simulink model "RoboSoccer"
settings: Solver=ode15s  StartTime=0.0  StopTime=inf  RelTol=1e-3
PreLoadFcn:
  | load busobjects.mat;
libraries: simulink x5
settings Model: Creator=smahapat  LastModifiedBy=user
settings SolverCC: ZeroCrossControl=DisableAll
settings DataIOCC: LimitDataPoints=on  SaveFormat=Array  SignalLoggingSaveFormat=ModelDataLogs  ReturnWorkspaceOutputs=off
settings OptimizationCC: InlineParams=on  ExpressionDepthLimit=2147483647  LifeSpan=inf  SimCompilerOptimization=Off
settings DebuggingCC: UnderspecifiedInitializationDetection=Classic  MergeDetectMultiDrivingBlocksExec=none  SolverPrmCheckMsg=warning  FcnCallInpInsideContextMsg=Use local settings  FrameProcessingCompatibilityMsg=warning  StateNameClashWarn=warning  SFUnexpectedBacktrackingDiag=warning  SFNoUnconditionalDefaultTransitionDiag=warning
settings HardwareCC: ProdBitPerPointer=32  ProdLargestAtomicFloat=None  ProdIntDivRoundTo=Undefined  ProdEndianess=Unspecified  ProdWordSize=32  ProdHWDeviceType=32-bit Generic
settings ModelReferenceCC: PropagateSignalLabelsOutOfModel=off
settings SFSimCC: SimUseLocalCustomCode=off  SimParseCustomCode=off
settings RTWCC: RTWUseLocalCustomCode=off  RTWCompilerOptimization=Off
settings CodeAppCC: CustomSymbolStrType=$N$R$M
settings GRTTargetCC: CodeReplacementLibrary=ANSI_C  GeneratePreprocessorConditionals=Disable all  CombineOutputUpdateFcns=off  CPPClassGenCompliant=off  GRTInterface=on

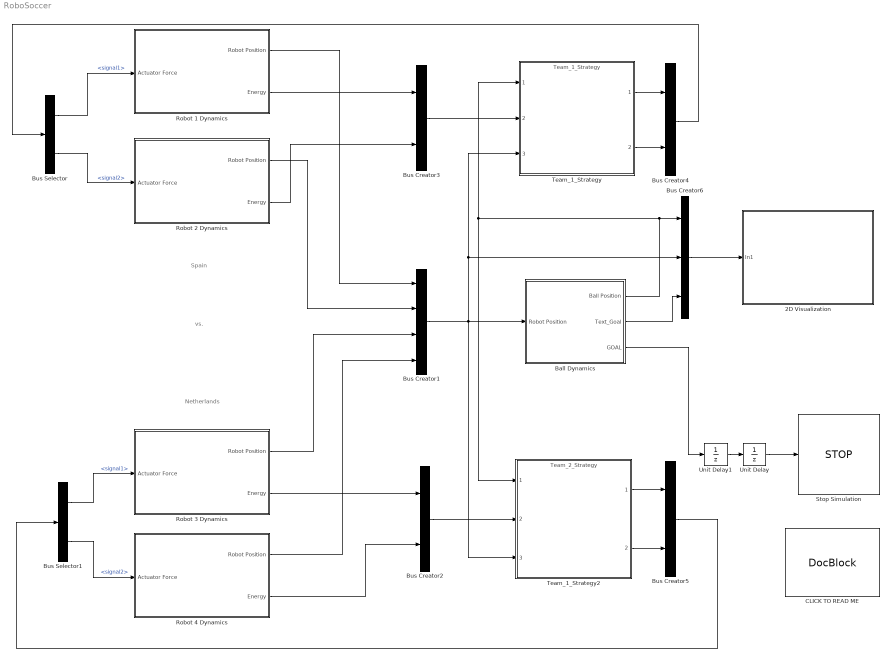
== system RoboSoccer ==
  note: Netherlands
  note: Spain
  note: vs.
  2D Visualization : Subsystem
      mask Display: image(imread('texture\3D_visualization.jpg'));
  Ball Dynamics : Subsystem  TreatAsAtomicUnit=on
      mask Display: image(imread('texture\soccer_ball_dynamics.jpg'));
  Bus Creator1 : BusCreator
  Bus Creator{2..5} (4 alike) : BusCreator  Inputs=2
  Bus Creator6 : BusCreator  Inputs=3
  Bus Selector : BusSelector  OutputSignals=signal1,signal2
  Bus Selector1 : BusSelector  OutputSignals=signal1,signal2
  CLICK TO READ ME : simulink/Model-Wide Utilities/DocBlock  DocumentType=Text
      content=|
      | Notes and help:
      | 1. The demo simulates a 2 vs. 2 robot scenario. The robots are assumed to be heavier than the football. Thus,
      | any collision between the ball and the robots is perfectly elastic. The robot motion is not impacted by the
      | collision.
      |
      | 2. Collision among robots is not implemented as they are considered as point masses.
      |
      | 3. Collision modeling in all cases is assumed to be as a spring contact model. When the object colliding with
      | a boundary comes close to that boundary, a force proprtional to the negative of the "penetration distance" is
      | computed.
      |
      | 4. The strategy subsystems are implemented as model references. This was done intentionally so that
      | competing teams could protect their strategies and run the simulation against each other. Use the model
      | protected mode to generate mdlp files instead of mdl files:
      |
      | >> Simulink.ModelReference.protect('Team_1_Strategy')
      |
      | and
      |
      | >> Simulink.ModelReference.protect('Team_2_Strategy')
      |
      | 5. Robot dynamics are simple dynamics of a point mass. However, the mass is inversely proportional to the
      | battery power or "stamina" of the robot. Some damping is also put into the system to avoid too much
      | overshoot. Also, each time the robot actuates itself or brakes, it incurs a small power loss thereby
      | lowering its endurance in the game.
      |
      | 6. Positional coordinates in the system are 2D i.e. (x,y). The signal dimensions have been set explicitly.
      | Click on any of the output ports->signal attributes of the masked subsystems to see the dimensions.
      |
      | 7. Ball dynamics has a simple implementation- same "spring-based" contact dynamics. From the ball's
      | point of view, there are five contact forces to be accounted for: contacts with the 4 robots and those of
      | the boundaries.
      |
      | 8. Observe that the solver has been changed to ode15s which is a stiff solver. The reason for this is
      | the stiffness present in the system because of the contact/collision modeling with high spring constants.
      | This can give rise to modes with relatively different dynamics. With a ode45 solver, the faster modes
      | will force the adaptive solver to take smaller steps slowing the simulation down. ode15s ignores some of
      | these fast dynamics.
      |
      | 9. All the icon drawing commands on the robot dynamics were implemented using the patch commands. These
      | were taken from the demo by Mike Woodward:
      |
      | http://www.mathworks.com/matlabcentral/fileexchange/8856-flags
      |
      | Use other flags to customize this.
      |
      | 10. 2D animation was done using Simulink 3D Animation. The field was textured with a grass image and a
      | viewpoint was so selected so that it looked as 2D. The "GOAL" text was kept behind the field. The moment,
      | a goal is scored, this text kis translated to the front giving a TV effect. Texturing was also used to
      | paint the bodies of the robots with the flags. You will have to change the images in order to change
      | these.
      |
      | 11. Play around with the strategy subsystems to see if you can come up with efficient strategies to score
      | early. Note that each of the teams has full knowledge of the others' positions and those of the ball. They
      | also have knowledge of the remaining power in their team's batteries. There is no velocity information
      | available.
      |
      | Questions:
      | 1. How can you use Stateflow to implement a fine state machine that uses a mix of attack and defensive
      | strategies based on ball location?
      |
      | 2. What block in Simulink should you use to input a new signal into these strategy subsystems so that
      | time elapsed since the start of the game can be measured and hence used as part of the strategy.
      |
      | 3. Identify the contents inside the MAT file used in the demo. What is the "type" of the contents of the
      | data inside the file? Identify the function that loads this MAT file.
      |
      | 4. Why did we need these data objects that you identified in 14 for our model?
      |
      | 5. Identify a model architecture that supports a 2n vs 2n game scenario ('n' is a natural number)
      |
      |
      |
      | 16.
  Robot 1 Dynamics : Subsystem  mask(Robot Parameters){P=0.5, saturate_value=0}
      mask prompts: P "Stamina (Enter value between 0 and 1)"; saturate_value "Actuator_saturation"
      mask help:
      | Set the robot stamina to a value between 0.1 and 1. Note that a higher value of stamina corresponds to more battery power which inversely impacts the mass of the robot. This will reduce its agility.
      |
      | Likewise, higher values of accuracy will come at a cost of higher rates of discharge for the battery pack.
      |
      | Choose values carefully to reflect these tradeoffs.
      mask init:
      | saturate_value=300;
      settings: CloseFcn=|
      | if P<0
      |     error('P cannot be less than 0');
      | end
      | if P>1
      |     error('P cannot be greater than 1');
      | end
      | 
      | if sigma<0
      |     error('sigma cannot be less than 0');
      | end
      | 
      | if sigma>1
      |     error('sigma cannot be greater than 1');
      | end
      mask Help:
      | Set the robot stamina to a value between 0.1 and 1. Note that a higher value of stamina corresponds to more battery power which inversely impacts the mass of the robot. This will reduce its agility.
      | 
      | Likewise, higher values of accuracy will come at a cost of higher rates of discharge for the battery pack.
      | 
      | Choose values carefully to reflect these tradeoffs.
      mask CallbackString: |saturate_value=10;
      mask Display:
      | patch([0 1 1 0], [0.75 0.75 1   1  ], [1 0 0]);
      | patch([0 1 1 0], [0.25 0.25 0.75 0.75], [1 1 0]);
      | patch([0 1 1 0], [0   0   0.25 0.25], [1 0 0]);
  Robot 2 Dynamics : Subsystem  mask(Robot Parameters){P=0.5, saturate_value=0}
      mask prompts: P "Stamina (Enter value between 0 and 1)"; saturate_value "Actuator_saturation"
      mask help:
      | Set the robot stamina to a value between 0.1 and 1. Note that a higher value of stamina corresponds to more battery power which inversely impacts the mass of the robot. This will reduce its agility.
      |
      | Likewise, higher values of accuracy will come at a cost of higher rates of discharge for the battery pack.
      |
      | Choose values carefully to reflect these tradeoffs.
      mask init:
      | saturate_value=300;
      settings: CloseFcn=|
      | if P<0
      |     error('P cannot be less than 0');
      | end
      | if P>1
      |     error('P cannot be greater than 1');
      | end
      | 
      | if sigma<0
      |     error('sigma cannot be less than 0');
      | end
      | 
      | if sigma>1
      |     error('sigma cannot be greater than 1');
      | end
      mask Help:
      | Set the robot stamina to a value between 0.1 and 1. Note that a higher value of stamina corresponds to more battery power which inversely impacts the mass of the robot. This will reduce its agility.
      | 
      | Likewise, higher values of accuracy will come at a cost of higher rates of discharge for the battery pack.
      | 
      | Choose values carefully to reflect these tradeoffs.
      mask CallbackString: |saturate_value=10;
      mask Display:
      | patch([0 1 1 0], [0.75 0.75 1   1  ], [1 0 0]);
      | patch([0 1 1 0], [0.25 0.25 0.75 0.75], [1 1 0]);
      | patch([0 1 1 0], [0   0   0.25 0.25], [1 0 0]);
  Robot 3 Dynamics : Subsystem  mask(Robot Parameters){P=0.5, saturate_value=0}
      mask prompts: P "Stamina (Enter value between 0 and 1)"; saturate_value "Actuator_saturation"
      mask help:
      | Set the robot stamina to a value between 0.1 and 1. Note that a higher value of stamina corresponds to more battery power which inversely impacts the mass of the robot. This will reduce its agility.
      |
      | Likewise, higher values of accuracy will come at a cost of higher rates of discharge for the battery pack.
      |
      | Choose values carefully to reflect these tradeoffs.
      mask init:
      | saturate_value=300;
      settings: CloseFcn=|
      | if P<0
      |     error('P cannot be less than 0');
      | end
      | if P>1
      |     error('P cannot be greater than 1');
      | end
      | 
      | if sigma<0
      |     error('sigma cannot be less than 0');
      | end
      | 
      | if sigma>1
      |     error('sigma cannot be greater than 1');
      | end
      mask Help:
      | Set the robot stamina to a value between 0.1 and 1. Note that a higher value of stamina corresponds to more battery power which inversely impacts the mass of the robot. This will reduce its agility.
      | 
      | Likewise, higher values of accuracy will come at a cost of higher rates of discharge for the battery pack.
      | 
      | Choose values carefully to reflect these tradeoffs.
      mask CallbackString: |saturate_value=10;
      mask Display:
      | patch([0 1 1 0], [2/3 2/3 1   1  ], [1 0 0]);
      | patch([0 1 1 0], [0   0   1/3 1/3], [0 0 1]);
  Robot 4 Dynamics : Subsystem  mask(Robot Parameters){P=0.5, saturate_value=0}
      mask prompts: P "Stamina (Enter value between 0 and 1)"; saturate_value "Actuator_saturation"
      mask help:
      | Set the robot stamina to a value between 0.1 and 1. Note that a higher value of stamina corresponds to more battery power which inversely impacts the mass of the robot. This will reduce its agility.
      |
      | Likewise, higher values of accuracy will come at a cost of higher rates of discharge for the battery pack.
      |
      | Choose values carefully to reflect these tradeoffs.
      mask init:
      | saturate_value=300;
      settings: CloseFcn=|
      | if P<0
      |     error('P cannot be less than 0');
      | end
      | if P>1
      |     error('P cannot be greater than 1');
      | end
      | 
      | if sigma<0
      |     error('sigma cannot be less than 0');
      | end
      | 
      | if sigma>1
      |     error('sigma cannot be greater than 1');
      | end
      mask Help:
      | Set the robot stamina to a value between 0.1 and 1. Note that a higher value of stamina corresponds to more battery power which inversely impacts the mass of the robot. This will reduce its agility.
      | 
      | Likewise, higher values of accuracy will come at a cost of higher rates of discharge for the battery pack.
      | 
      | Choose values carefully to reflect these tradeoffs.
      mask CallbackString: |saturate_value=10;
      mask Display:
      | patch([0 1 1 0], [2/3 2/3 1   1  ], [1 0 0]);
      | patch([0 1 1 0], [0   0   1/3 1/3], [0 0 1]);
  Stop Simulation : Stop
  Team_1_Strategy : ModelReference  ModelNameDialog=Team_1_Strategy  SimulationMode=Normal  ModelReferenceVersion=1.30  CopyOfModelName=Team_1_Strategy  DefaultDataLogging=off
      mask Display:
      | disp(' TEAM 1\n\n')
      | disp('STRATEGY')
  Team_1_Strategy2 : ModelReference  ModelNameDialog=Team_2_Strategy  SimulationMode=Normal  ModelReferenceVersion=1.28  CopyOfModelName=Team_2_Strategy  DefaultDataLogging=off
      mask Display:
      | disp(' TEAM 2\n\n')
      | disp('STRATEGY')
  Unit Delay : UnitDelay  SampleTime=-1
  Unit Delay1 : UnitDelay  SampleTime=-1
  wires:
  Robot 1 Dynamics/1(Robot Position) -> Bus Creator1/1
  Robot 2 Dynamics/1(Robot Position) -> Bus Creator1/2
  Robot 3 Dynamics/1(Robot Position) -> Bus Creator1/3
  Robot 4 Dynamics/1(Robot Position) -> Bus Creator1/4
  Bus Creator1/1 -> Ball Dynamics/1(Robot Position), Bus Creator6/2, Team_1_Strategy/3, Team_1_Strategy2/3
  Robot 3 Dynamics/2(Energy) -> Bus Creator2/1
  Robot 4 Dynamics/2(Energy) -> Bus Creator2/2
  Bus Creator2/1 -> Team_1_Strategy2/2
  Team_1_Strategy2/1 -> Bus Creator5/1
  Team_1_Strategy2/2 -> Bus Creator5/2
  Bus Creator5/1 -> Bus Selector1/1
  Team_1_Strategy/1 -> Bus Creator4/1
  Team_1_Strategy/2 -> Bus Creator4/2
  Bus Creator4/1 -> Bus Selector/1
  Bus Selector/1 -> Robot 1 Dynamics/1(Actuator Force)  "<signal1>"
  Bus Selector/2 -> Robot 2 Dynamics/1(Actuator Force)  "<signal2>"
  Bus Selector1/1 -> Robot 3 Dynamics/1(Actuator Force)  "<signal1>"
  Bus Selector1/2 -> Robot 4 Dynamics/1(Actuator Force)  "<signal2>"
  Ball Dynamics/3(GOAL) -> Unit Delay1/1
  Ball Dynamics/1(Ball Position) -> Bus Creator6/1, Team_1_Strategy/1, Team_1_Strategy2/1
  Bus Creator6/1 -> 2D Visualization/1(In1)
  Ball Dynamics/2(Text_Goal) -> Bus Creator6/3
  Bus Creator3/1 -> Team_1_Strategy/2
  Robot 2 Dynamics/2(Energy) -> Bus Creator3/2
  Robot 1 Dynamics/2(Energy) -> Bus Creator3/1
  Unit Delay/1 -> Stop Simulation/1
  Unit Delay1/1 -> Unit Delay/1

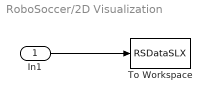
== system RoboSoccer/2D Visualization ==
  In1 : Inport
  To Workspace : ToWorkspace  VariableName=RSDataSLX  SampleTime=-1
  wires:
  In1/1 -> To Workspace/1

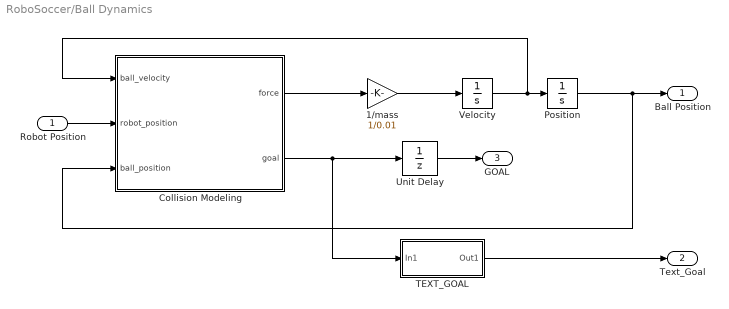
== system RoboSoccer/Ball Dynamics ==
  Robot Position : Inport
  1/mass : Gain  Gain=1/0.01
  Collision Modeling : MATLAB Function  TreatAsAtomicUnit=on
  Position : Integrator  InitialCondition=[100;50]
  TEXT_GOAL : Subsystem
  Unit Delay : UnitDelay  SampleTime=-1
  Velocity : Integrator  InitialCondition=[0;0]
  Ball Position : Outport
  Text_Goal : Outport  Port=2
  GOAL : Outport  Port=3
  wires:
  Robot Position/1 -> Collision Modeling/2(robot_position)
  Velocity/1 -> Position/1, Collision Modeling/1(ball_velocity)
  Position/1 -> Ball Position/1, Collision Modeling/3(ball_position)
  Collision Modeling/1(force) -> 1/mass/1
  1/mass/1 -> Velocity/1
  Collision Modeling/2(goal) -> Unit Delay/1, TEXT_GOAL/1(In1)
  Unit Delay/1 -> GOAL/1
  TEXT_GOAL/1(Out1) -> Text_Goal/1

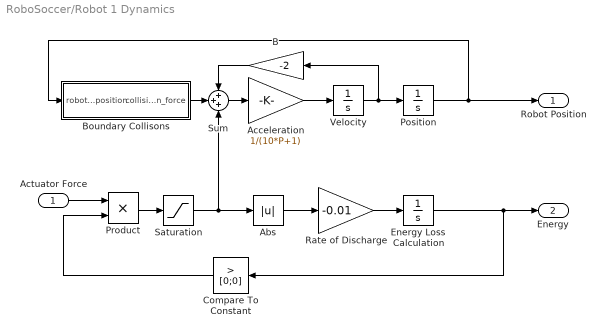
== system RoboSoccer/Robot 1 Dynamics ==
  Actuator Force : Inport
  Abs : Abs
  Acceleration : Gain  Gain=1/(10*P+1)
  B : Gain  Gain=-2
  Boundary Collisons : MATLAB Function  TreatAsAtomicUnit=on
  Compare To Constant : simulink/Logic and Bit Operations/Compare To Constant  relop=>  const=[0;0]  OutDataTypeStr=uint8
  Energy Loss Calculation : Integrator  InitialCondition=1000*[P; P]
  Position : Integrator  InitialCondition=[50; 75]
  Product : Product  RndMeth=Zero
  Rate of Discharge : Gain  Gain=-0.01
  Saturation : Saturate  UpperLimit=saturate_value  LowerLimit=-saturate_value
  Sum : Sum  Inputs=+++
  Velocity : Integrator  InitialCondition=[0;0]
  Robot Position : Outport  PortDimensions=[2 1]
  Energy : Outport  Port=2  PortDimensions=[2 1]
  wires:
  Acceleration/1 -> Velocity/1
  Velocity/1 -> Position/1, B/1
  Position/1 -> Boundary Collisons/1(robot_position), Robot Position/1
  Energy Loss Calculation/1 -> Energy/1, Compare To Constant/1
  Rate of Discharge/1 -> Energy Loss Calculation/1
  Saturation/1 -> Abs/1, Sum/3
  Abs/1 -> Rate of Discharge/1
  Actuator Force/1 -> Product/1
  Product/1 -> Saturation/1
  Compare To Constant/1 -> Product/2
  Boundary Collisons/1(collision_force) -> Sum/2
  Sum/1 -> Acceleration/1
  B/1 -> Sum/1

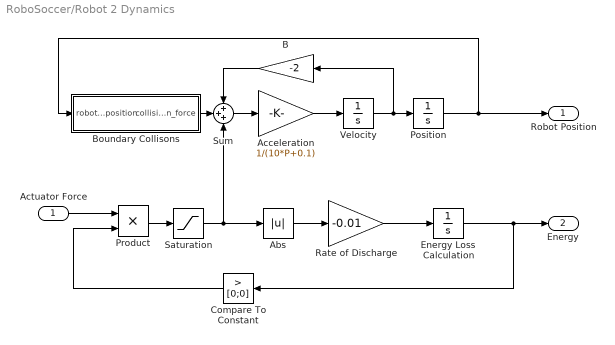
== system RoboSoccer/Robot 2 Dynamics ==
  Actuator Force : Inport
  Abs : Abs
  Acceleration : Gain  Gain=1/(10*P+0.1)
  B : Gain  Gain=-2
  Boundary Collisons : MATLAB Function  TreatAsAtomicUnit=on
  Compare To Constant : simulink/Logic and Bit Operations/Compare To Constant  relop=>  const=[0;0]  OutDataTypeStr=uint8
  Energy Loss Calculation : Integrator  InitialCondition=1000*[P; P]
  Position : Integrator  InitialCondition=[50; 25]
  Product : Product  RndMeth=Zero
  Rate of Discharge : Gain  Gain=-0.01
  Saturation : Saturate  UpperLimit=saturate_value  LowerLimit=-saturate_value
  Sum : Sum  Inputs=+++
  Velocity : Integrator  InitialCondition=[0;0]
  Robot Position : Outport  PortDimensions=[2 1]
  Energy : Outport  Port=2  PortDimensions=[2 1]
  wires:
  Compare To Constant/1 -> Product/2
  Product/1 -> Saturation/1
  Actuator Force/1 -> Product/1
  Abs/1 -> Rate of Discharge/1
  Saturation/1 -> Abs/1, Sum/3
  Rate of Discharge/1 -> Energy Loss Calculation/1
  Energy Loss Calculation/1 -> Compare To Constant/1, Energy/1
  Position/1 -> Robot Position/1, Boundary Collisons/1(robot_position)
  Velocity/1 -> Position/1, B/1
  Acceleration/1 -> Velocity/1
  Sum/1 -> Acceleration/1
  Boundary Collisons/1(collision_force) -> Sum/2
  B/1 -> Sum/1

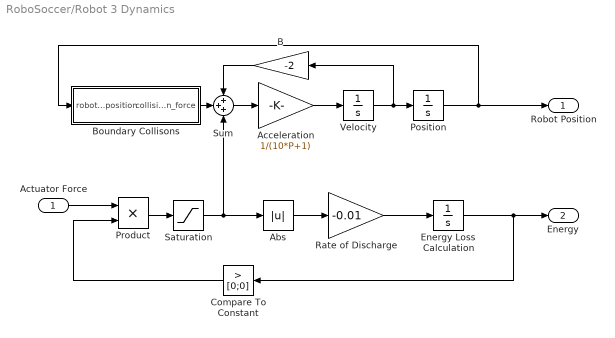
== system RoboSoccer/Robot 3 Dynamics ==
  Actuator Force : Inport
  Abs : Abs
  Acceleration : Gain  Gain=1/(10*P+1)
  B : Gain  Gain=-2
  Boundary Collisons : MATLAB Function  TreatAsAtomicUnit=on
  Compare To Constant : simulink/Logic and Bit Operations/Compare To Constant  relop=>  const=[0;0]  OutDataTypeStr=uint8
  Energy Loss Calculation : Integrator  InitialCondition=1000*[P; P]
  Position : Integrator  InitialCondition=[150; 75]
  Product : Product  RndMeth=Zero
  Rate of Discharge : Gain  Gain=-0.01
  Saturation : Saturate  UpperLimit=saturate_value  LowerLimit=-saturate_value
  Sum : Sum  Inputs=+++
  Velocity : Integrator  InitialCondition=[0;0]
  Robot Position : Outport  PortDimensions=[2 1]
  Energy : Outport  Port=2  PortDimensions=[2 1]
  wires:
  Compare To Constant/1 -> Product/2
  Product/1 -> Saturation/1
  Actuator Force/1 -> Product/1
  Abs/1 -> Rate of Discharge/1
  Saturation/1 -> Abs/1, Sum/3
  Rate of Discharge/1 -> Energy Loss Calculation/1
  Energy Loss Calculation/1 -> Compare To Constant/1, Energy/1
  Position/1 -> Robot Position/1, Boundary Collisons/1(robot_position)
  Velocity/1 -> Position/1, B/1
  Acceleration/1 -> Velocity/1
  Sum/1 -> Acceleration/1
  Boundary Collisons/1(collision_force) -> Sum/2
  B/1 -> Sum/1

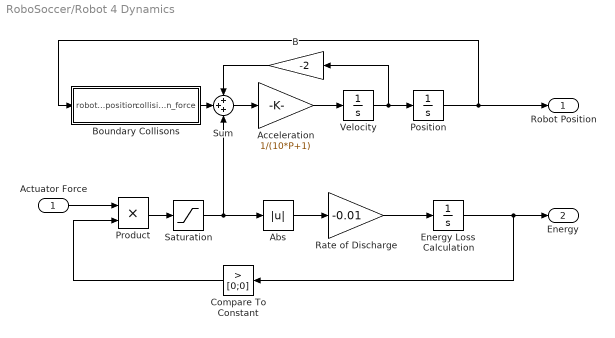
== system RoboSoccer/Robot 4 Dynamics ==
  Actuator Force : Inport
  Abs : Abs
  Acceleration : Gain  Gain=1/(10*P+1)
  B : Gain  Gain=-2
  Boundary Collisons : MATLAB Function  TreatAsAtomicUnit=on
  Compare To Constant : simulink/Logic and Bit Operations/Compare To Constant  relop=>  const=[0;0]  OutDataTypeStr=uint8
  Energy Loss Calculation : Integrator  InitialCondition=1000*[P; P]
  Position : Integrator  InitialCondition=[150; 25]
  Product : Product  RndMeth=Zero
  Rate of Discharge : Gain  Gain=-0.01
  Saturation : Saturate  UpperLimit=saturate_value  LowerLimit=-saturate_value
  Sum : Sum  Inputs=+++
  Velocity : Integrator  InitialCondition=[0;0]
  Robot Position : Outport  PortDimensions=[2 1]
  Energy : Outport  Port=2  PortDimensions=[2 1]
  wires:
  Sum/1 -> Acceleration/1
  Acceleration/1 -> Velocity/1
  Velocity/1 -> Position/1, B/1
  Position/1 -> Boundary Collisons/1(robot_position), Robot Position/1
  Energy Loss Calculation/1 -> Energy/1, Compare To Constant/1
  Rate of Discharge/1 -> Energy Loss Calculation/1
  Saturation/1 -> Abs/1, Sum/3
  Abs/1 -> Rate of Discharge/1
  Actuator Force/1 -> Product/1
  Product/1 -> Saturation/1
  Compare To Constant/1 -> Product/2
  Boundary Collisons/1(collision_force) -> Sum/2
  B/1 -> Sum/1

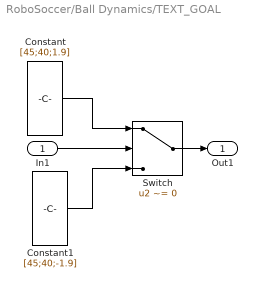
== system RoboSoccer/Ball Dynamics/TEXT_GOAL ==
  In1 : Inport
  Constant : Constant  Value=[45;40;1.9]
  Constant1 : Constant  Value=[45;40;-1.9]
  Switch : Switch  Criteria=u2 ~= 0  Threshold=1
  Out1 : Outport
  wires:
  In1/1 -> Switch/2
  Switch/1 -> Out1/1
  Constant/1 -> Switch/1
  Constant1/1 -> Switch/3

== matlab function RoboSoccer/Ball Dynamics/Collision Modeling ==
  data: ball_velocity input; robot_position input size=[8 ;1]; ball_position input size=[2;1]; force output size=[2;1]; goal output
function [force, goal] = fcn(ball_velocity,robot_position, ball_position)
%#eml
% Initialize variables

force1=zeros(2,1);
force2=zeros(2,1);
force3=zeros(2,1);
force4=zeros(2,1);
collision_force=zeros(2,1);
d1=zeros(2,1);
d2=zeros(2,1);
d3=zeros(2,1);
d4=zeros(2,1);
K=100;
goal=0;
tol=25;
B=0.01;

% Compute dot products and calculate impulsive forces on the ball
d1=robot_position(1:2,1)-ball_position;
d2=robot_position(3:4,1)-ball_position;
d3=robot_position(5:6,1)-ball_position;
d4=robot_position(7:8,1)-ball_position;

if   dot(d1,d1) <tol
     force1=-K*d1;
end

if   dot(d2,d2) <tol
     force2=-K*d2;
end

if   dot(d3,d3) <tol
     force3=-K*d3;
end

if   dot(d4,d4) <tol
     force4=-K*d4;
end

% Code to check for boundary collisions for the ball
if ball_position(1,1)<0 
    collision_force(1,1)=-K*ball_position(1,1);
end

if ball_position(1,1)>200 
    collision_force(1,1)=K*(200-ball_position(1,1));
end

if ball_position(2,1)<0 
    collision_force(2,1)=-K*ball_position(2,1);
end

if ball_position(2,1)>100 
    collision_force(2,1)=K*(100-ball_position(2,1)); 
end

% Total force
force=collision_force+force1+force2+force3+force4-B*ball_velocity;

% Goal scored
if ((ball_position(1,1)<=0) && (ball_position(2,1)>41) && (ball_position(2,1)<59))
    goal=1; 
end

if ((ball_position(1,1)>=200) && (ball_position(2,1)>41) && (ball_position(2,1)<59))
    goal=1; 
end

== matlab function RoboSoccer/Robot 1 Dynamics/Boundary Collisons ==
  data: robot_position input; collision_force output
function collision_force = fcn(robot_position)
%#eml
K=100;
collision_force=[0; 0]; 
if robot_position(1,1)<0 
    collision_force(1,1)=-K*robot_position(1,1);
end

if robot_position(1,1)>200 
    collision_force(1,1)=K*(200-robot_position(1,1));
end

if robot_position(2,1)<0 
    collision_force(2,1)=-K*robot_position(2,1);
end

if robot_position(2,1)>100 
    collision_force(2,1)=K*(100-robot_position(2,1));
end

== matlab function RoboSoccer/Robot 4 Dynamics/Boundary Collisons ==
  data: robot_position input; collision_force output
function collision_force = fcn(robot_position)
%#eml
K=100;
collision_force=[0; 0]; 
if robot_position(1,1)<0 
    collision_force(1,1)=-K*robot_position(1,1);
end

if robot_position(1,1)>200 
    collision_force(1,1)=K*(200-robot_position(1,1));
end

if robot_position(2,1)<0 
    collision_force(2,1)=-K*robot_position(2,1);
end

if robot_position(2,1)>100 
    collision_force(2,1)=K*(100-robot_position(2,1));
end

== matlab function RoboSoccer/Robot 3 Dynamics/Boundary Collisons ==
  data: robot_position input; collision_force output
function collision_force = fcn(robot_position)
%#eml
K=100;
collision_force=[0; 0]; 
if robot_position(1,1)<0 
    collision_force(1,1)=-K*robot_position(1,1);
end

if robot_position(1,1)>200 
    collision_force(1,1)=K*(200-robot_position(1,1));
end

if robot_position(2,1)<0 
    collision_force(2,1)=-K*robot_position(2,1);
end

if robot_position(2,1)>100 
    collision_force(2,1)=K*(100-robot_position(2,1));
end

== matlab function RoboSoccer/Robot 2 Dynamics/Boundary Collisons ==
  data: robot_position input; collision_force output
function collision_force = fcn(robot_position)
%#eml
K=100;
collision_force=[0; 0]; 
if robot_position(1,1)<0 
    collision_force(1,1)=-K*robot_position(1,1);
end

if robot_position(1,1)>200 
    collision_force(1,1)=K*(200-robot_position(1,1));
end

if robot_position(2,1)<0 
    collision_force(2,1)=-K*robot_position(2,1);
end

if robot_position(2,1)>100 
    collision_force(2,1)=K*(100-robot_position(2,1));
end
